simulink model "sim_system_lin_retour_etat_aug"  (Simulink 8.1)
settings: Solver=ode3  StartTime=0.0  StopTime=t_simu  FixedStep=0.020  RelTol=1e-3
values from neighbouring files (symbols this model uses):
  A_lin_a = [A_lin [0 0 0]' ; 0 0 1 0]    [main.m]    (also in retour_etat_augmente.m)
  B_lin_a = [B_lin ; 0 0]    [main.m]    (also in retour_etat_augmente.m)
  C_charge_max = f_ctl(Wf_max + Wf_0, Ng_0) - C_charge_0    [main.m]    (also in retour_etat_augmente.m)
  C_charge_min = f_ctl(Wf_min + Wf_0, Ng_0) - C_charge_0    [main.m]    (also in retour_etat_augmente.m)
  C_lin_a = [C_lin [0 0 0 0]' ; 0 0 0 1]    [main.m]    (also in retour_etat_augmente.m)
  D_lin_a = [D_lin ; 0 0]    [main.m]    (also in retour_etat_augmente.m)
  dWf_max = 100    [main.m]    (also in retour_etat_augmente.m)
  K_feedback_2_aug = place(A_lin_a, B_lin_a(:,1), poles_goal_aug)    [main.m]    (also in retour_etat_augmente.m)
  ss_capteur_temperature = ss(A_capteur_temperature, B_capteur_temperature, C_capteur_temperature, D_capteur_temperature)    [ss_doseur_capteur.m]
  T45_0 = f_t45(Wf_0, Ng_0)    [point_equilibre.m]
  t_step = t_simu / 2    (= 50)    [main.m]    (also in retour_etat_augmente.m; retour_etat_simple.m = 12.5)
  Wf_max = f_wfmax(P3_0) - Wf_0    [main.m]    (also in retour_etat_augmente.m)
  Wf_min = 60 - Wf_0    [main.m]    (also in retour_etat_augmente.m)
settings Model: Creator=maffre  LastModifiedBy=martinpetrov
settings DebuggingCC: FcnCallInpInsideContextMsg=EnableAllAsWarning

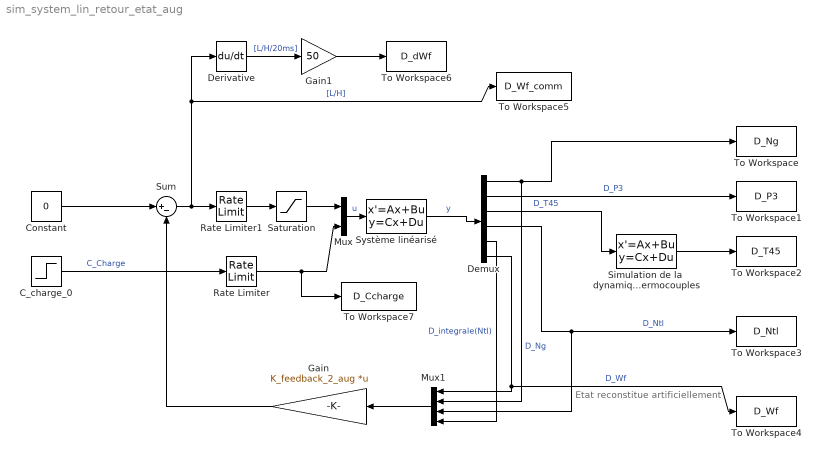
== system sim_system_lin_retour_etat_aug ==
  note: Etat reconstitue artificiellement
  C_charge_0 : Step  Time=t_step  Before=C_charge_min  After=C_charge_max  SampleTime=0
  Constant : Constant  Value=0
  Demux : Demux  Outputs=6
  Derivative : Derivative
  Gain : Gain  Gain=K_feedback_2_aug  Multiplication=Matrix(K*u)
  Gain1 : Gain  Gain=50
  Mux : Mux  Inputs=2
  Mux1 : Mux
  Rate Limiter : RateLimiter  RisingSlewLimit=64  FallingSlewLimit=-64  SampleTimeMode=inherited
  Rate Limiter1 : RateLimiter  RisingSlewLimit=dWf_max  FallingSlewLimit=-dWf_max  SampleTimeMode=inherited
  Saturation : Saturate  UpperLimit=Wf_max  LowerLimit=Wf_min
  Simulation de la  dynamique des  thermocouples : StateSpace  A=ss_capteur_temperature.A  B=ss_capteur_temperature.B  C=ss_capteur_temperature.C  D=ss_capteur_temperature.D  X0=T45_0
  Sum : Sum  Inputs=|+-
  Système linéarisé : StateSpace  A=A_lin_a  B=B_lin_a  C=[C_lin_a ; 1 0 0 0]  D=[D_lin_a ; 0 0]
  To Workspace : ToWorkspace  VariableName=D_Ng  SampleTime=-1  SaveFormat=Structure With Time
  To Workspace1 : ToWorkspace  VariableName=D_P3  SampleTime=-1  SaveFormat=Structure With Time
  To Workspace2 : ToWorkspace  VariableName=D_T45  SampleTime=-1  SaveFormat=Structure With Time
  To Workspace3 : ToWorkspace  VariableName=D_Ntl  SampleTime=-1  SaveFormat=Structure With Time
  To Workspace4 : ToWorkspace  VariableName=D_Wf  SampleTime=-1  SaveFormat=Structure With Time
  To Workspace5 : ToWorkspace  VariableName=D_Wf_comm  SampleTime=-1  SaveFormat=Structure With Time
  To Workspace6 : ToWorkspace  VariableName=D_dWf  SampleTime=-1  SaveFormat=Structure With Time
  To Workspace7 : ToWorkspace  VariableName=D_Ccharge  SampleTime=-1  SaveFormat=Structure With Time
  wires:
  Système linéarisé/1 -> Demux/1  "y"
  Demux/1 -> To Workspace/1, Mux1/2  "D_Ng"
  Demux/2 -> To Workspace1/1  "D_P3"
  Demux/4 -> To Workspace3/1, Mux1/3  "D_Ntl"
  Mux/1 -> Système linéarisé/1  "u"
  Simulation de la  dynamique des  thermocouples/1 -> To Workspace2/1
  Demux/3 -> Simulation de la  dynamique des  thermocouples/1  "D_T45"
  Mux1/1 -> Gain/1
  Sum/1 -> Derivative/1, To Workspace5/1, Rate Limiter1/1  "[L/H]"
  Gain/1 -> Sum/2
  Constant/1 -> Sum/1
  Demux/6 -> To Workspace4/1, Mux1/1  "D_Wf"
  Demux/5 -> Mux1/4  "D_integrale(Ntl)"
  Gain1/1 -> To Workspace6/1
  Derivative/1 -> Gain1/1  "[L/H/20ms]"
  Rate Limiter/1 -> To Workspace7/1, Mux/2
  C_charge_0/1 -> Rate Limiter/1  "C_Charge"
  Rate Limiter1/1 -> Saturation/1
  Saturation/1 -> Mux/1
